simulink model "Wind_dist_lat"  (R2021a)
settings: Solver=VariableStepAuto  StartTime=0.0  StopTime=5  MinStep=0.0001  RelTol=1e-10  AbsTol=1e-10
undefined symbols (not defined in the file): A, B, B1
libraries: dspsrcs4 x2
settings Model: Creator=Lenovo  LastModifiedBy=Lenovo
settings SolverCC: InitialStep=0.01

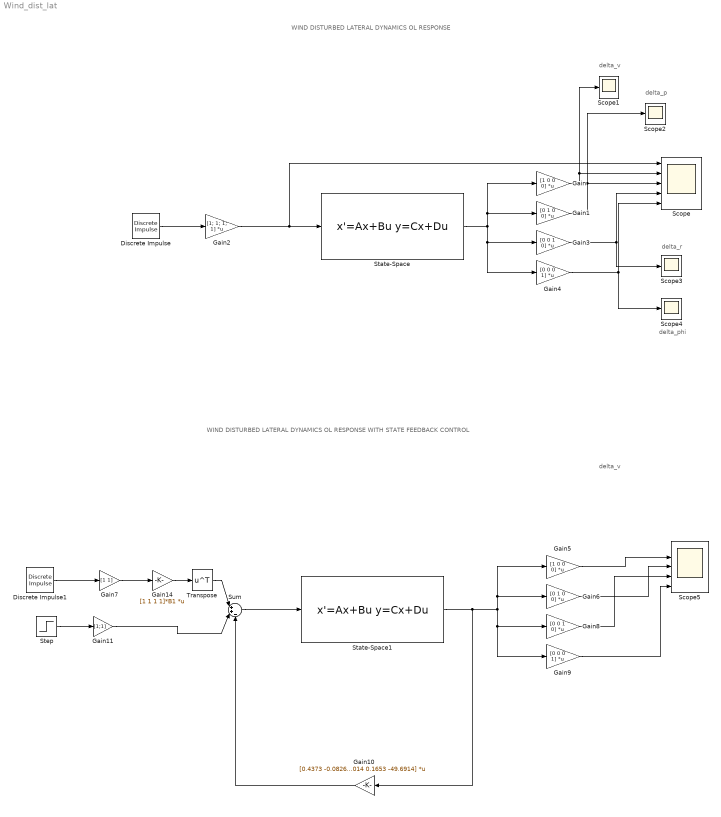
== system Wind_dist_lat ==
  note: delta_phi
  note: delta_r
  note: delta_p
  note: delta_v
  note: WIND DISTURBED LATERAL DYNAMICS OL RESPONSE WITH STATE FEEDBACK CONTROL
  note: WIND DISTURBED LATERAL DYNAMICS OL RESPONSE
  note: delta_v
  Discrete Impulse : dspsrcs4/Discrete  Impulse  Delay=0  SampleTime=1  FrameSample=1  OutputFrames=off  dataType=double  isSigned=on  wordLen=16  udDataType=sfix(16)  fracBitsMode=Best precision  numFracBits=15  OutDataTypeStr=double  LastOutDataTypeStr=double
  Discrete Impulse1 : dspsrcs4/Discrete  Impulse  Delay=0  SampleTime=1  FrameSample=1  OutputFrames=off  dataType=double  isSigned=on  wordLen=16  udDataType=sfix(16)  fracBitsMode=Best precision  numFracBits=15  OutDataTypeStr=double  LastOutDataTypeStr=double
  Gain : Gain  Gain=[1 0 0 0]  Multiplication=Matrix(K*u)
  Gain1 : Gain  Gain=[0 1 0 0]  Multiplication=Matrix(K*u)
  Gain10 : Gain  Gain=[0.4373 -0.0826 0.5153 4.3401; -0.0495 -0.6014 0.1653 -49.6914]  Multiplication=Matrix(K*u)
  Gain11 : Gain  Gain=[1;1]
  Gain14 : Gain  Gain=[1 1 1 1]*B1  Multiplication=Matrix(K*u) (u vector)
  Gain2 : Gain  Gain=[1; 1; 1; 1]  Multiplication=Matrix(K*u)
  Gain3 : Gain  Gain=[0 0 1 0]  Multiplication=Matrix(K*u)
  Gain4 : Gain  Gain=[0 0 0 1]  Multiplication=Matrix(K*u)
  Gain5 : Gain  Gain=[1 0 0 0]  Multiplication=Matrix(K*u)
  Gain6 : Gain  Gain=[0 1 0 0]  Multiplication=Matrix(K*u)
  Gain7 : Gain  Gain=[1 1]
  Gain8 : Gain  Gain=[0 0 1 0]  Multiplication=Matrix(K*u)
  Gain9 : Gain  Gain=[0 0 0 1]  Multiplication=Matrix(K*u)
  Scope : Scope  NumInputPorts=5
  Scope{1..4} (4 alike) : Scope
  Scope5 : Scope  NumInputPorts=5
  State-Space : StateSpace  A=[-0.0869 0 -1 0.039; -4.424 -1.184 0.335 0; 2.148 -0.021 -0.228 0; 0 1 0 0]  B=[0.0223 0 0.0869 0; 0.547 2.12 4.424 1.184; -1.169 0.065 0 -1; 0 0 -2.148 0.21]  C=[1 0 0 0;0 1 0 0;0 0 1 0;0 0 0 1]  D=[0 0 0 0; 0 0 0 0; 0 0 0 0; 0 0 0 0]  InitialCondition=0
  State-Space1 : StateSpace  A=A  B=B  C=[1 0 0 0;0 1 0 0; 0 0 1 0; 0 0 0 1]  D=zeros(4,2)  InitialCondition=0  ParameterTunability=Optimized
  Step : Step  Time=0  After=0.2  SampleTime=0
  Sum : Sum  Inputs=|++-
  Transpose : Math  Operator=transpose  SaturateOnIntegerOverflow=on
  wires:
  State-Space1/1 -> Gain10/1, Gain6/1, Gain5/1, Gain9/1, Gain8/1
  Discrete Impulse/1 -> Gain2/1
  Gain4/1 -> Scope4/1, Scope/5
  Gain3/1 -> Scope3/1, Scope/4
  State-Space/1 -> Gain1/1, Gain/1, Gain4/1, Gain3/1
  Gain1/1 -> Scope2/1, Scope/3
  Gain/1 -> Scope1/1, Scope/2
  Gain2/1 -> Scope/1, State-Space/1
  Transpose/1 -> Sum/1
  Gain14/1 -> Transpose/1
  Discrete Impulse1/1 -> Gain7/1
  Gain7/1 -> Gain14/1
  Gain11/1 -> Sum/2
  Sum/1 -> State-Space1/1
  Step/1 -> Gain11/1
  Gain10/1 -> Sum/3
  Gain5/1 -> Scope5/2
  Gain6/1 -> Scope5/3
  Gain8/1 -> Scope5/4
  Gain9/1 -> Scope5/5
